simulink model "inv_rot_pen_RL_swingup_2_train"  (R2025b)
settings: Solver=FixedStepAuto  StartTime=0.0  StopTime=1  FixedStep=Ts  RelTol=1e-3
StopFcn:
  | myStopFcnAppendInitTime
values from neighbouring files (symbols this model uses):
  cfg = loaded.cfg    [continueFurutaMatlabSwingupTraining.m]    (also in evaluateFurutaController.m = makeFurutaConfig(); evaluateFurutaMatlabSwingupAgent.m = makeFurutaMatlabSwingupTD3Config(); finalizeFurutaDirectTD3Run.m = normalizeRunConfig(cfg, runDir); initFurutaSldrtHardwareWorkspace.m = makeFurutaMathWorksStyleWideTD3Config())
  i_max = 4    [initFurutaModelWorkspace.m]
  K = K_oben    [initFurutaModelWorkspace.m]
  Kp_i = db2mag(options.CurrentControllerKpDb)    [initFurutaModelWorkspace.m]    (also in initFurutaSldrtHardwareWorkspace.m = 2.5)
  omega0 = options.InitialOmega    [initFurutaModelWorkspace.m]
  param = get_parameter()    [initFurutaModelWorkspace.m]
  s = zpk("s")    [initFurutaModelWorkspace.m]    (also in initFurutaSldrtHardwareWorkspace.m)
  theta0 = options.InitialTheta    [initFurutaModelWorkspace.m]
  Tn_i = param.L / param.R    [initFurutaModelWorkspace.m]    (also in initFurutaSldrtHardwareWorkspace.m = 0.000286849073257)
undefined symbols (not defined in the file or in its folder): doneParams, rewardParams, safetyParams, X, Y, Z
libraries: sm_lib x19, nesl_utility x6, rllib x2, simulink x1
settings Model: SimulationMode=accelerator  Creator=abuj  LastModifiedBy=abuj
settings DataIOCC: SaveOutput=off  DSMLogging=off  SaveTime=off  ReturnWorkspaceOutputs=off
settings ExplorerConfigSet: SimMechanicsOpenEditorOnUpdate=off

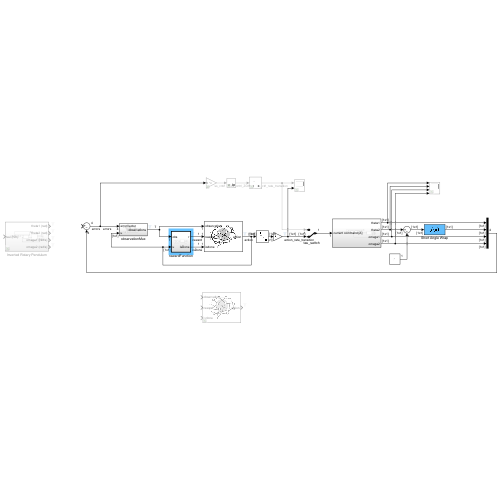
[thumbnail: Simulink's stored preview of the top-level diagram]
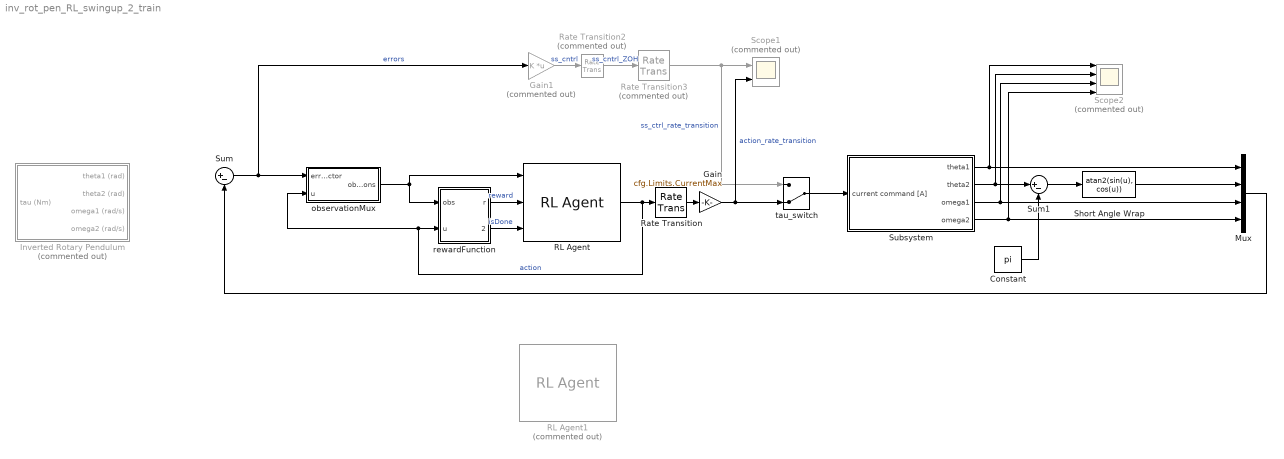
== system inv_rot_pen_RL_swingup_2_train ==
  Constant : Constant  Value=pi
  Gain : Gain  Gain=cfg.Limits.CurrentMax
  Gain1 : Gain  Commented=on  Gain=K  Multiplication=Matrix(K*u)
  Inverted Rotary Pendulum : Subsystem  Commented=on
  Mux : Mux
  RL Agent : rllib/RL Agent  Agent=agent  ExternalActionAsInput=off  ProvideLastAction=off  ProvideCumRwd=off  TreatAsDirectFeedthrough=on  UseStrictObservationDataTypes=off
  RL Agent1 : rllib/RL Agent  Commented=on  Agent=agent  ExternalActionAsInput=off  ProvideLastAction=off  ProvideCumRwd=off  TreatAsDirectFeedthrough=on  UseStrictObservationDataTypes=off
  Rate Transition : RateTransition  OutPortSampleTime=Ts
  Rate Transition2 : RateTransition  Commented=on  OutPortSampleTime=cfg.Agent.SampleTime
  Rate Transition3 : RateTransition  Commented=on  OutPortSampleTime=Ts
  Scope1 : Scope  Commented=on  NumInputPorts=2
      settings: ActiveDisplayYMinimum=-4.2971254580337988  ActiveDisplayYMaximum=0.512065850784593  DataLoggingVariableName=ScopeData4
  Scope2 : Scope  Commented=on  NumInputPorts=4
      settings: ActiveDisplayYMinimum=-1.667283029169482  ActiveDisplayYMaximum=0.18527228980949279
  Short Angle Wrap : Fcn  Expr=atan2(sin(u), cos(u))
  Subsystem : Subsystem
  Sum : Sum  Inputs=|+-
  Sum1 : Sum  Inputs=|+-
  observationMux : Subsystem
  rewardFunction : Subsystem  TreatAsAtomicUnit=on  SystemSampleTime=cfg.Agent.SampleTime
  tau_switch : ManualSwitch  CurrentSetting=0
  wires:
  Sum1/1 -> Short Angle Wrap/1
  Constant/1 -> Sum1/2
  Mux/1 -> Sum/2
  Rate Transition/1 -> Gain/1
  Subsystem/4(omega2) -> Scope2/4, Mux/4
  Subsystem/1(theta1) -> Scope2/1, Mux/1
  Subsystem/2(theta2) -> Scope2/2, Sum1/1
  Subsystem/3(omega1) -> Scope2/3, Mux/3
  Short Angle Wrap/1 -> Mux/2
  Gain1/1 -> Rate Transition2/1  "ss_cntrl"
  Rate Transition2/1 -> Rate Transition3/1  "ss_cntrl_ZOH"
  Rate Transition3/1 -> Scope1/1, tau_switch/1  "ss_ctrl_rate_transition"
  tau_switch/1 -> Subsystem/1(current command [A])
  Gain/1 -> Scope1/2, tau_switch/2  "action_rate_transition"
  rewardFunction/1(r) -> RL Agent/2  "reward"
  Sum/1 -> observationMux/1(errorVector), Gain1/1  "errors"
  rewardFunction/2(isDone) -> RL Agent/3  "isDone"
  RL Agent/1 -> rewardFunction/2(u), observationMux/2(u), Rate Transition/1  "action"
  observationMux/1(observations) -> rewardFunction/1(obs), RL Agent/1

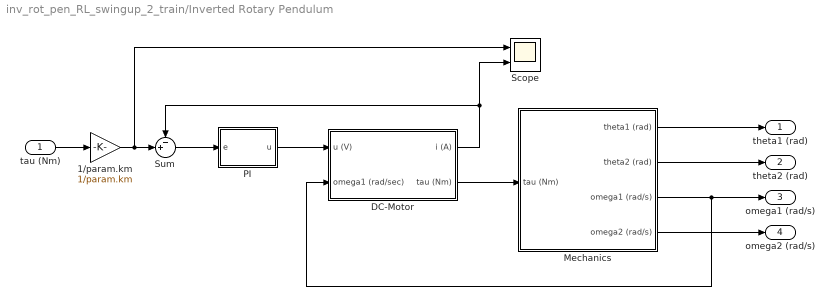
== system inv_rot_pen_RL_swingup_2_train/Inverted Rotary Pendulum ==
  tau (Nm) : Inport
  1/param.km : Gain  Gain=1/param.km
  DC-Motor : Subsystem
  Mechanics : Subsystem
  PI : Subsystem
  Scope : Scope  NumInputPorts=2
      settings: ActiveDisplayYMinimum=-0.091534229828850844  ActiveDisplayYMaximum=0.52735330073349629  DataLoggingVariableName=ScopeData2
  Sum : Sum  Inputs=-+|
  theta1 (rad) : Outport
  theta2 (rad) : Outport  Port=2
  omega1 (rad/s) : Outport  Port=3
  omega2 (rad/s) : Outport  Port=4
  wires:
  Mechanics/1(theta1 (rad)) -> theta1 (rad)/1
  Mechanics/2(theta2 (rad)) -> theta2 (rad)/1
  Mechanics/3(omega1 (rad/s)) -> DC-Motor/2(omega1 (rad/sec)), omega1 (rad/s)/1
  Mechanics/4(omega2 (rad/s)) -> omega2 (rad/s)/1
  DC-Motor/2(tau (Nm)) -> Mechanics/1(tau (Nm))
  Sum/1 -> PI/1(e)
  PI/1(u) -> DC-Motor/1(u (V))
  DC-Motor/1(i (A)) -> Scope/2, Sum/1
  tau (Nm)/1 -> 1/param.km/1
  1/param.km/1 -> Scope/1, Sum/2

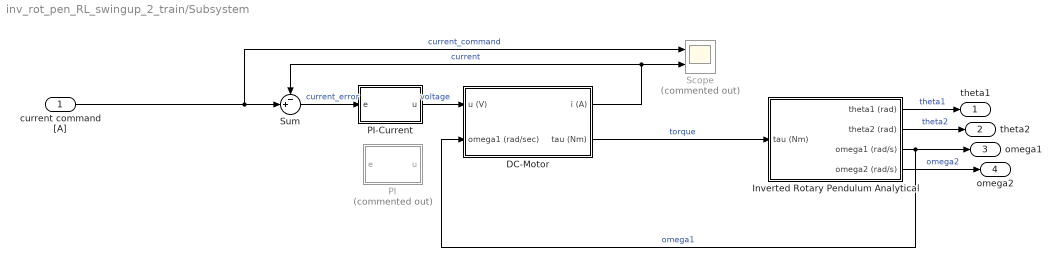
== system inv_rot_pen_RL_swingup_2_train/Subsystem ==
  current command [A] : Inport
  DC-Motor : Subsystem
  Inverted Rotary Pendulum Analytical : Subsystem
  PI : Subsystem  Commented=on
  PI-Current : Subsystem
  Scope : Scope  Commented=on  NumInputPorts=2
      settings: ActiveDisplayYMinimum=-4.5  ActiveDisplayYMaximum=0.49999999999999989
  Sum : Sum  Inputs=-+|
  theta1 : Outport
  theta2 : Outport  Port=2
  omega1 : Outport  Port=3
  omega2 : Outport  Port=4
  wires:
  Inverted Rotary Pendulum Analytical/3(omega1 (rad/s)) -> omega1/1, DC-Motor/2(omega1 (rad/sec))  "omega1"
  Inverted Rotary Pendulum Analytical/1(theta1 (rad)) -> theta1/1  "theta1"
  Inverted Rotary Pendulum Analytical/4(omega2 (rad/s)) -> omega2/1  "omega2"
  Inverted Rotary Pendulum Analytical/2(theta2 (rad)) -> theta2/1  "theta2"
  PI-Current/1(u) -> DC-Motor/1(u (V))  "voltage"
  DC-Motor/2(tau (Nm)) -> Inverted Rotary Pendulum Analytical/1(tau (Nm))  "torque"
  current command [A]/1 -> Scope/1, Sum/2  "current_command"
  DC-Motor/1(i (A)) -> Sum/1, Scope/2  "current"
  Sum/1 -> PI-Current/1(e)  "current_error"

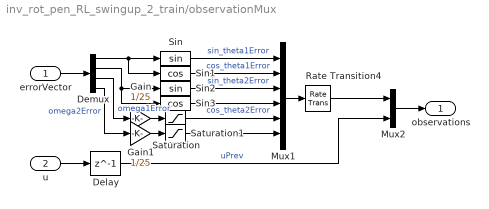
== system inv_rot_pen_RL_swingup_2_train/observationMux ==
  errorVector : Inport
  u : Inport  Port=2
  Delay : Delay  DelayLength=1
  Demux : Demux
  Gain : Gain  Gain=1/25
  Gain1 : Gain  Gain=1/25
  Mux1 : Mux  Inputs=6
  Mux2 : Mux  Inputs=2
  Rate Transition4 : RateTransition  OutPortSampleTime=cfg.Agent.SampleTime
  Saturation : Saturate  UpperLimit=25  LowerLimit=-25
  Saturation1 : Saturate  UpperLimit=25  LowerLimit=-25
  Sin : Trigonometry
  Sin1 : Trigonometry  Operator=cos
  Sin2 : Trigonometry
  Sin3 : Trigonometry  Operator=cos
  observations : Outport
  wires:
  Demux/2 -> Sin3/1, Sin2/1
  Sin1/1 -> Mux1/2  "cos_theta1Error"
  Demux/1 -> Sin1/1, Sin/1
  Rate Transition4/1 -> Mux2/1
  Mux1/1 -> Rate Transition4/1
  Sin/1 -> Mux1/1  "sin_theta1Error"
  Sin3/1 -> Mux1/4  "cos_theta2Error"
  errorVector/1 -> Demux/1
  Demux/4 -> Gain1/1  "omega2Error"
  Demux/3 -> Gain/1  "omega1Error"
  Sin2/1 -> Mux1/3  "sin_theta2Error"
  Mux2/1 -> observations/1
  u/1 -> Delay/1
  Delay/1 -> Mux2/2  "uPrev"
  Gain/1 -> Saturation/1
  Saturation/1 -> Mux1/5
  Gain1/1 -> Saturation1/1
  Saturation1/1 -> Mux1/6

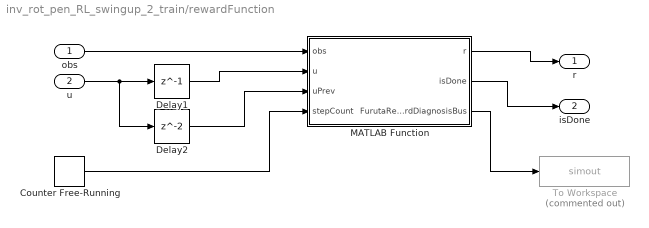
== system inv_rot_pen_RL_swingup_2_train/rewardFunction ==
  obs : Inport
  u : Inport  Port=2
  Counter Free-Running : simulink/Sources/Counter Free-Running  NumBits=16  tsamp=-1
  Delay1 : Delay  DelayLength=1  SampleTime=cfg.Agent.SampleTime
  Delay2 : Delay  SampleTime=cfg.Agent.SampleTime
  MATLAB Function : MATLAB Function  TreatAsAtomicUnit=on
  To Workspace : ToWorkspace  Commented=on  VariableName=simout  SaveFormat=Timeseries  SampleTime=-1
  r : Outport
  isDone : Outport  Port=2
  wires:
  MATLAB Function/2(isDone) -> isDone/1
  obs/1 -> MATLAB Function/1(obs)
  MATLAB Function/1(r) -> r/1
  u/1 -> Delay2/1, Delay1/1
  Delay2/1 -> MATLAB Function/3(uPrev)
  Delay1/1 -> MATLAB Function/2(u)
  MATLAB Function/3(FurutaRewardDiagnosisBus) -> To Workspace/1
  Counter Free-Running/1 -> MATLAB Function/4(stepCount)

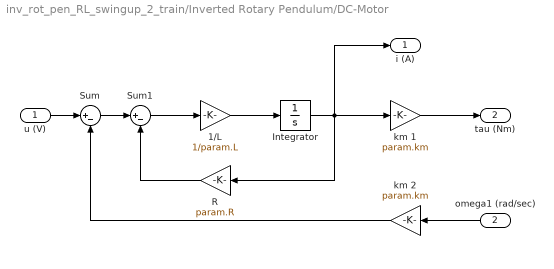
== system inv_rot_pen_RL_swingup_2_train/Inverted Rotary Pendulum/DC-Motor ==
  u (V) : Inport
  omega1 (rad/sec) : Inport  Port=2
  1/L : Gain  Gain=1/param.L
  Integrator : Integrator
  R : Gain  Gain=param.R
  Sum : Sum  Inputs=|+-
  Sum1 : Sum  Inputs=|+-
  km 1 : Gain  Gain=param.km
  km 2 : Gain  Gain=param.km
  i (A) : Outport
  tau (Nm) : Outport  Port=2
  wires:
  R/1 -> Sum1/2
  Integrator/1 -> i (A)/1, km 1/1, R/1
  u (V)/1 -> Sum/1
  Sum1/1 -> 1/L/1
  Sum/1 -> Sum1/1
  1/L/1 -> Integrator/1
  omega1 (rad/sec)/1 -> km 2/1
  km 2/1 -> Sum/2
  km 1/1 -> tau (Nm)/1

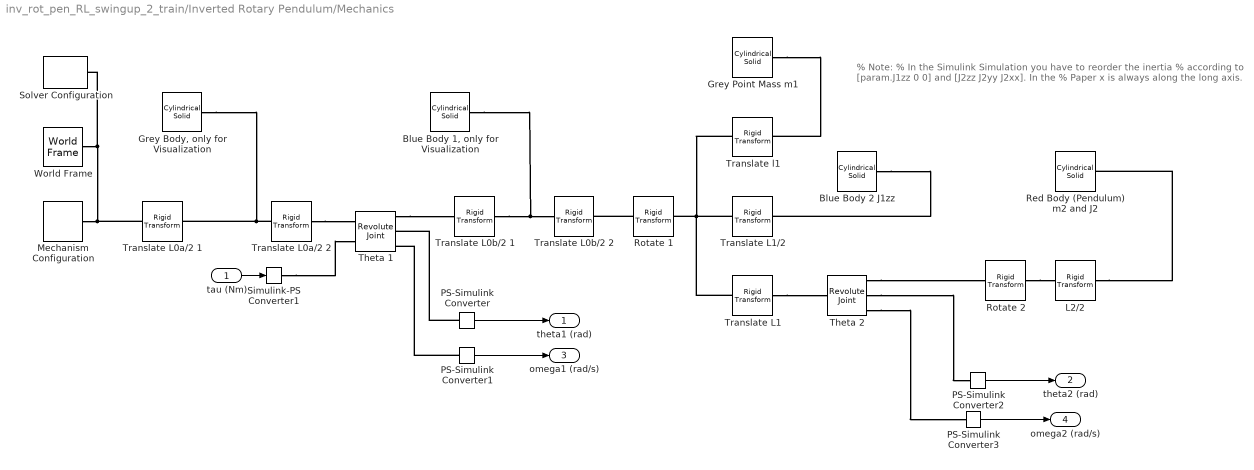
== system inv_rot_pen_RL_swingup_2_train/Inverted Rotary Pendulum/Mechanics ==
  note: % Note:
      | % In the Simulink Simulation you have to reorder the inertia
      | % according to [param.J1zz 0 0] and [J2zz J2yy J2xx]. In the
      | % Paper x is always along the long axis.
  tau (Nm) : Inport
  "Blue Body 1, only for Visualization" : sm_lib/Body Elements/Cylindrical Solid  CylinderRadius=param.r0b  CylinderRadiusUnits=m  CylinderLength=param.L0b  CylinderLengthUnits=m  ExportEntireGeometry=off  InertiaType=PointMass  BasedOnType=Density  Density=1000  DensityUnits=kg/m^3  Mass=0  MassUnits=kg  CenterOfMass=[0 0 0]  CenterOfMassUnits=m  MomentsOfInertia=[0 0 0]  MomentsOfInertiaUnits=kg*m^2  ProductsOfInertia=[0 0 0]  ProductsOfInertiaUnits=kg*m^2  GraphicType=FromGeometry  MarkerShape=Sphere  MarkerSize=10  GraphicVisPropType=SimpleVisualProperties  GraphicDiffuseColor=[0.0 0.6 1.0]  GraphicOpacity=1  GraphicSpecularColor=[0.5 0.5 0.5 1.0]  GraphicAmbientColor=[0.15 0.15 0.15 1.0]  GraphicEmissiveColor=[0.0 0.0 0.0 1.0]  GraphicShininess=75  DoExposeReferenceFrame=on  SerializedFrames=<Frames/>
  Blue Body 2 J1zz : sm_lib/Body Elements/Cylindrical Solid  CylinderRadius=param.r1  CylinderRadiusUnits=m  CylinderLength=param.L1  CylinderLengthUnits=m  ExportEntireGeometry=off  InertiaType=Custom  BasedOnType=Density  Density=1000  DensityUnits=kg/m^3  Mass=0  MassUnits=kg  CenterOfMass=[0 0 0]  CenterOfMassUnits=m  MomentsOfInertia=[param.J1zz 0 0]  MomentsOfInertiaUnits=kg*m^2  ProductsOfInertia=[0 0 0]  ProductsOfInertiaUnits=kg*m^2  GraphicType=FromGeometry  MarkerShape=Sphere  MarkerSize=10  GraphicVisPropType=SimpleVisualProperties  GraphicDiffuseColor=[0.0 0.6 1.0]  GraphicOpacity=1  GraphicSpecularColor=[0.5 0.5 0.5 1.0]  GraphicAmbientColor=[0.15 0.15 0.15 1.0]  GraphicEmissiveColor=[0.0 0.0 0.0 1.0]  GraphicShininess=75  DoExposeReferenceFrame=on  SerializedFrames=<Frames/>
  "Grey Body, only for Visualization" : sm_lib/Body Elements/Cylindrical Solid  CylinderRadius=param.r0a  CylinderRadiusUnits=m  CylinderLength=param.L0a  CylinderLengthUnits=m  ExportEntireGeometry=off  InertiaType=PointMass  BasedOnType=Density  Density=1000  DensityUnits=kg/m^3  Mass=0  MassUnits=kg  CenterOfMass=[0 0 0]  CenterOfMassUnits=m  MomentsOfInertia=[0 0 0]  MomentsOfInertiaUnits=kg*m^2  ProductsOfInertia=[0 0 0]  ProductsOfInertiaUnits=kg*m^2  GraphicType=FromGeometry  MarkerShape=Sphere  MarkerSize=10  GraphicVisPropType=SimpleVisualProperties  GraphicDiffuseColor=[0.5 0.5 0.5]  GraphicOpacity=1  GraphicSpecularColor=[0.5 0.5 0.5 1.0]  GraphicAmbientColor=[0.15 0.15 0.15 1.0]  GraphicEmissiveColor=[0.0 0.0 0.0 1.0]  GraphicShininess=75  DoExposeReferenceFrame=on  SerializedFrames=<Frames/>
  Grey Point Mass m1 : sm_lib/Body Elements/Cylindrical Solid  CylinderRadius=1  CylinderRadiusUnits=m  CylinderLength=1  CylinderLengthUnits=m  ExportEntireGeometry=off  InertiaType=PointMass  BasedOnType=Density  Density=1000  DensityUnits=kg/m^3  Mass=param.m1  MassUnits=kg  CenterOfMass=[0 0 0]  CenterOfMassUnits=m  MomentsOfInertia=[1 1 1]  MomentsOfInertiaUnits=kg*m^2  ProductsOfInertia=[0 0 0]  ProductsOfInertiaUnits=kg*m^2  GraphicType=Marker  MarkerShape=Sphere  MarkerSize=10  GraphicVisPropType=SimpleVisualProperties  GraphicDiffuseColor=[0.5 0.5 0.5]  GraphicOpacity=1  GraphicSpecularColor=[0.5 0.5 0.5 1.0]  GraphicAmbientColor=[0.15 0.15 0.15 1.0]  GraphicEmissiveColor=[0.0 0.0 0.0 1.0]  GraphicShininess=75  DoExposeReferenceFrame=on  SerializedFrames=<Frames/>
  L2/2 : sm_lib/Frames and Transforms/Rigid Transform  RotationMethod=None  FollAlignAxisA=+X  BaseAlignAxisA=+Y  FollAlignAxisB=+Y  BaseAlignAxisB=+Z  RotationStandardAxis=+Z  RotationAngle=0  RotationAngleUnits=deg  RotationArbitraryAxis=[0 0 1]  RotationSequenceAxes=FollowerAxes  RotationSequence=ZYX  RotationSequenceAngles=[0 pi/2 0]  RotationSequenceAnglesUnits=rad  RotationMatrix=[1 0 0;0 1 0;0 0 1]  Quaternion=[1 0 0 0]  TranslationMethod=Cartesian  TranslationCartesianOffset=[0 0 param.L2/2]  TranslationCartesianOffsetUnits=m  TranslationStandardAxis=+Z  TranslationStandardOffset=0  TranslationStandardOffsetUnits=m  TranslationROffset=0  TranslationROffsetUnits=m  TranslationThetaOffset=0  TranslationThetaOffsetUnits=deg  TranslationZOffset=0  TranslationZOffsetUnits=m
  Mechanism Configuration : sm_lib/Utilities/Mechanism Configuration  UniformGravity=Constant  GravityVector=[0 0 -param.g]  GravityVectorUnits=m/s^2  LinearizationDelta=0.001  JointModeTransitionNonlinearIterations=2
  PS-Simulink Converter{,1..3} (4 alike) : nesl_utility/PS-Simulink Converter  PhysicalDomain=network_engine_domain  SubClassName=ps_output  LeftPortType=input  RightPortType=output  PseudoPeriodic=off  Frequencies=[]  VectorFormat=inherit  Unit=inherit  AffineConversion=off
  Red Body (Pendulum) m2 and J2 : sm_lib/Body Elements/Cylindrical Solid  CylinderRadius=param.r2  CylinderRadiusUnits=m  CylinderLength=param.L2  CylinderLengthUnits=m  ExportEntireGeometry=off  InertiaType=Custom  BasedOnType=Density  Density=1000  DensityUnits=kg/m^3  Mass=param.m2  MassUnits=kg  CenterOfMass=[0 0 0]  CenterOfMassUnits=m  MomentsOfInertia=[param.J2zz param.J2yy param.J2xx]  MomentsOfInertiaUnits=kg*m^2  ProductsOfInertia=[0 0 0]  ProductsOfInertiaUnits=kg*m^2  GraphicType=FromGeometry  MarkerShape=Sphere  MarkerSize=10  GraphicVisPropType=SimpleVisualProperties  GraphicDiffuseColor=[1.0 0.2 0.2]  GraphicOpacity=1  GraphicSpecularColor=[0.5 0.5 0.5 1.0]  GraphicAmbientColor=[0.15 0.15 0.15 1.0]  GraphicEmissiveColor=[0.0 0.0 0.0 1.0]  GraphicShininess=75  DoExposeReferenceFrame=on  SerializedFrames=<Frames/>
  Rotate 1 : sm_lib/Frames and Transforms/Rigid Transform  RotationMethod=RotationSequence  FollAlignAxisA=+X  BaseAlignAxisA=+Y  FollAlignAxisB=+Y  BaseAlignAxisB=+Z  RotationStandardAxis=+Z  RotationAngle=0  RotationAngleUnits=deg  RotationArbitraryAxis=[0 0 1]  RotationSequenceAxes=FollowerAxes  RotationSequence=ZYX  RotationSequenceAngles=[0 pi/2 0]  RotationSequenceAnglesUnits=rad  RotationMatrix=[1 0 0;0 1 0;0 0 1]  Quaternion=[1 0 0 0]  TranslationMethod=None  TranslationCartesianOffset=[0 0 0]  TranslationCartesianOffsetUnits=m  TranslationStandardAxis=+Z  TranslationStandardOffset=0  TranslationStandardOffsetUnits=m  TranslationROffset=0  TranslationROffsetUnits=m  TranslationThetaOffset=0  TranslationThetaOffsetUnits=deg  TranslationZOffset=0  TranslationZOffsetUnits=m
  Rotate 2 : sm_lib/Frames and Transforms/Rigid Transform  RotationMethod=RotationSequence  FollAlignAxisA=+X  BaseAlignAxisA=+Y  FollAlignAxisB=+Y  BaseAlignAxisB=+Z  RotationStandardAxis=+Z  RotationAngle=0  RotationAngleUnits=deg  RotationArbitraryAxis=[0 0 1]  RotationSequenceAxes=FollowerAxes  RotationSequence=ZYX  RotationSequenceAngles=[0 pi/2 0]  RotationSequenceAnglesUnits=rad  RotationMatrix=[1 0 0;0 1 0;0 0 1]  Quaternion=[1 0 0 0]  TranslationMethod=None  TranslationCartesianOffset=[0 0 0]  TranslationCartesianOffsetUnits=m  TranslationStandardAxis=+Z  TranslationStandardOffset=0  TranslationStandardOffsetUnits=m  TranslationROffset=0  TranslationROffsetUnits=m  TranslationThetaOffset=0  TranslationThetaOffsetUnits=deg  TranslationZOffset=0  TranslationZOffsetUnits=m
  Simulink-PS Converter1 : nesl_utility/Simulink-PS Converter  PhysicalDomain=network_engine_domain  SubClassName=ps_input  LeftPortType=input  RightPortType=output  PseudoPeriodic=off  Frequencies=[]  NoiseDistribution=none  NoiseParameters=[]  Unit=1  AffineConversion=off  FilteringAndDerivatives=provide  SimscapeFilterOrder=1  InputFilterTimeConstant=0.001  UdotUserProvided=0
  Solver Configuration : nesl_utility/Solver Configuration  PhysicalDomain=network_engine_domain  SubClassName=solver  LeftPortType=input  RightPortType=generic  Tones=[]  Harmonics=[]  SimulateNoise=off  Profile=off  UseLocalSampling=off  EnableSwitchedLinearOptims=on  FrequencyDomain=off  UseCCode=off  RelTol=0.001  AbsTol=0.001  MinStep=1e-09  ToWorkspace=off  RevertToSquareIcSolve=off  NumHomotopyIterations=100  PhasorMode=off  PhasorModeNumHarmonics=1  ConsistencySolver=NEWTON_XTOL_AFTER_FTOL  IndexReductionMethod=DerivativeReplacement  DoDC=off  ResidualTolerance=1e-09  ConsistencyTolSource=GLOBAL  ConsistencyAbsTol=0.001  ConsistencyRelTol=0.001  ConsistencyTolFactor=0.001  UseLocalSolver=off  LocalSolverChoice=NE_BACKWARD_EULER_ADVANCER  ResolveIndetEquations=on  FunctionEvalNumThread=1  LocalSolverSampleTime=0.001  DoFixedCost=off  MaxNonlinIter=3  MaxModeIter=2  ComputeImpulses=off  ImpulseIterations=2  LinearAlgebra=auto  LinearAlgebraNumThread=0  EquationFormulation=NE_TIME_EF  DelaysMemoryBudget=1024  AutomaticFiltering=on  FilteringTimeConstant=0.001  PartitionStorageMethod=AS_NEEDED  PartitionMemoryBudget=1024  PartitionMethod=ROBUST  MultibodyUseLocalSolver=off  MultibodyLocalSolverChoice=ODE1  MultibodyLocalSolverSampleTime=0.001
  Theta 1 : sm_lib/Joints/Revolute Joint  JointMode=Normal  CompositeWrenchDir=FollowerOnBase  CompositeWrenchFrame=BaseFrame  SenseConstraintForce=off  SenseConstraintTorque=off  SenseTotalForce=off  SenseTotalTorque=off  PositionTargetSpecify=on  PositionTargetPriority=High  PositionTargetValue=theta0(1)  PositionTargetValueUnits=rad  VelocityTargetSpecify=off  VelocityTargetPriority=High  VelocityTargetValue=0  VelocityTargetValueUnits=deg/s  EquilibriumPosition=0  EquilibriumPositionUnits=rad  SpringStiffness=0  SpringStiffnessUnits=N*m/rad  DampingCoefficient=param.b1  DampingCoefficientUnits=N*m*s/rad  LowerLimitSpecify=off  LowerLimitBound=-90  LowerLimitBoundUnits=deg  LowerLimitStiffness=1e4  LowerLimitStiffnessUnits=N*m/deg  LowerLimitDamping=10  LowerLimitDampingUnits=N*m/(deg/s)  LowerLimitTransitionRegionWidth=0.1  LowerLimitTransitionRegionWidthUnits=deg  UpperLimitSpecify=off  UpperLimitBound=90  UpperLimitBoundUnits=deg  UpperLimitStiffness=1e4  UpperLimitStiffnessUnits=N*m/deg  UpperLimitDamping=10  UpperLimitDampingUnits=N*m/(deg/s)  UpperLimitTransitionRegionWidth=0.1  UpperLimitTransitionRegionWidthUnits=deg  TorqueActuationMode=InputTorque  MotionActuationMode=ComputedMotion  SensePosition=on  SenseVelocity=on  SenseAcceleration=off  SenseTorqueForce=off  SenseLowerLimitTorqueForce=off  SenseUpperLimitTorqueForce=off
  Theta 2 : sm_lib/Joints/Revolute Joint  JointMode=Normal  CompositeWrenchDir=FollowerOnBase  CompositeWrenchFrame=BaseFrame  SenseConstraintForce=off  SenseConstraintTorque=off  SenseTotalForce=off  SenseTotalTorque=off  PositionTargetSpecify=on  PositionTargetPriority=High  PositionTargetValue=theta0(2)  PositionTargetValueUnits=rad  VelocityTargetSpecify=off  VelocityTargetPriority=High  VelocityTargetValue=0  VelocityTargetValueUnits=deg/s  EquilibriumPosition=0  EquilibriumPositionUnits=rad  SpringStiffness=0  SpringStiffnessUnits=N*m/rad  DampingCoefficient=param.b2  DampingCoefficientUnits=N*m*s/rad  LowerLimitSpecify=off  LowerLimitBound=-90  LowerLimitBoundUnits=deg  LowerLimitStiffness=1e4  LowerLimitStiffnessUnits=N*m/deg  LowerLimitDamping=10  LowerLimitDampingUnits=N*m/(deg/s)  LowerLimitTransitionRegionWidth=0.1  LowerLimitTransitionRegionWidthUnits=deg  UpperLimitSpecify=off  UpperLimitBound=90  UpperLimitBoundUnits=deg  UpperLimitStiffness=1e4  UpperLimitStiffnessUnits=N*m/deg  UpperLimitDamping=10  UpperLimitDampingUnits=N*m/(deg/s)  UpperLimitTransitionRegionWidth=0.1  UpperLimitTransitionRegionWidthUnits=deg  TorqueActuationMode=NoTorque  MotionActuationMode=ComputedMotion  SensePosition=on  SenseVelocity=on  SenseAcceleration=off  SenseTorqueForce=off  SenseLowerLimitTorqueForce=off  SenseUpperLimitTorqueForce=off
  Translate L0a/2 1 : sm_lib/Frames and Transforms/Rigid Transform  RotationMethod=None  FollAlignAxisA=+X  BaseAlignAxisA=+Y  FollAlignAxisB=+Y  BaseAlignAxisB=+Z  RotationStandardAxis=+Z  RotationAngle=0  RotationAngleUnits=deg  RotationArbitraryAxis=[0 0 1]  RotationSequenceAxes=FollowerAxes  RotationSequence=ZYX  RotationSequenceAngles=[0 0 0]  RotationSequenceAnglesUnits=rad  RotationMatrix=[1 0 0;0 1 0;0 0 1]  Quaternion=[1 0 0 0]  TranslationMethod=Cartesian  TranslationCartesianOffset=[0 0 param.L0a/2]  TranslationCartesianOffsetUnits=m  TranslationStandardAxis=+Z  TranslationStandardOffset=0  TranslationStandardOffsetUnits=m  TranslationROffset=0  TranslationROffsetUnits=m  TranslationThetaOffset=0  TranslationThetaOffsetUnits=deg  TranslationZOffset=0  TranslationZOffsetUnits=m
  Translate L0a/2 2 : sm_lib/Frames and Transforms/Rigid Transform  RotationMethod=None  FollAlignAxisA=+X  BaseAlignAxisA=+Y  FollAlignAxisB=+Y  BaseAlignAxisB=+Z  RotationStandardAxis=+Z  RotationAngle=0  RotationAngleUnits=deg  RotationArbitraryAxis=[0 0 1]  RotationSequenceAxes=FollowerAxes  RotationSequence=ZYX  RotationSequenceAngles=[0 0 0]  RotationSequenceAnglesUnits=rad  RotationMatrix=[1 0 0;0 1 0;0 0 1]  Quaternion=[1 0 0 0]  TranslationMethod=Cartesian  TranslationCartesianOffset=[0 0 param.L0a/2]  TranslationCartesianOffsetUnits=m  TranslationStandardAxis=+Z  TranslationStandardOffset=0  TranslationStandardOffsetUnits=m  TranslationROffset=0  TranslationROffsetUnits=m  TranslationThetaOffset=0  TranslationThetaOffsetUnits=deg  TranslationZOffset=0  TranslationZOffsetUnits=m
  Translate L0b/2 1 : sm_lib/Frames and Transforms/Rigid Transform  RotationMethod=None  FollAlignAxisA=+X  BaseAlignAxisA=+Y  FollAlignAxisB=+Y  BaseAlignAxisB=+Z  RotationStandardAxis=+Z  RotationAngle=0  RotationAngleUnits=deg  RotationArbitraryAxis=[0 0 1]  RotationSequenceAxes=FollowerAxes  RotationSequence=ZYX  RotationSequenceAngles=[0 0 0]  RotationSequenceAnglesUnits=rad  RotationMatrix=[1 0 0;0 1 0;0 0 1]  Quaternion=[1 0 0 0]  TranslationMethod=Cartesian  TranslationCartesianOffset=[0 0 param.L0b/2]  TranslationCartesianOffsetUnits=m  TranslationStandardAxis=+Z  TranslationStandardOffset=0  TranslationStandardOffsetUnits=m  TranslationROffset=0  TranslationROffsetUnits=m  TranslationThetaOffset=0  TranslationThetaOffsetUnits=deg  TranslationZOffset=0  TranslationZOffsetUnits=m
  Translate L0b/2 2 : sm_lib/Frames and Transforms/Rigid Transform  RotationMethod=None  FollAlignAxisA=+X  BaseAlignAxisA=+Y  FollAlignAxisB=+Y  BaseAlignAxisB=+Z  RotationStandardAxis=+Z  RotationAngle=0  RotationAngleUnits=deg  RotationArbitraryAxis=[0 0 1]  RotationSequenceAxes=FollowerAxes  RotationSequence=ZYX  RotationSequenceAngles=[0 0 0]  RotationSequenceAnglesUnits=rad  RotationMatrix=[1 0 0;0 1 0;0 0 1]  Quaternion=[1 0 0 0]  TranslationMethod=Cartesian  TranslationCartesianOffset=[0 0 param.L0b/2]  TranslationCartesianOffsetUnits=m  TranslationStandardAxis=+Z  TranslationStandardOffset=0  TranslationStandardOffsetUnits=m  TranslationROffset=0  TranslationROffsetUnits=m  TranslationThetaOffset=0  TranslationThetaOffsetUnits=deg  TranslationZOffset=0  TranslationZOffsetUnits=m
  Translate L1 : sm_lib/Frames and Transforms/Rigid Transform  RotationMethod=None  FollAlignAxisA=+X  BaseAlignAxisA=+Y  FollAlignAxisB=+Y  BaseAlignAxisB=+Z  RotationStandardAxis=+Z  RotationAngle=0  RotationAngleUnits=deg  RotationArbitraryAxis=[0 0 1]  RotationSequenceAxes=FollowerAxes  RotationSequence=ZYX  RotationSequenceAngles=[0 0 0]  RotationSequenceAnglesUnits=rad  RotationMatrix=[1 0 0;0 1 0;0 0 1]  Quaternion=[1 0 0 0]  TranslationMethod=Cartesian  TranslationCartesianOffset=[0 0 param.L1]  TranslationCartesianOffsetUnits=m  TranslationStandardAxis=+Z  TranslationStandardOffset=0  TranslationStandardOffsetUnits=m  TranslationROffset=0  TranslationROffsetUnits=m  TranslationThetaOffset=0  TranslationThetaOffsetUnits=deg  TranslationZOffset=0  TranslationZOffsetUnits=m
  Translate L1/2 : sm_lib/Frames and Transforms/Rigid Transform  RotationMethod=None  FollAlignAxisA=+X  BaseAlignAxisA=+Y  FollAlignAxisB=+Y  BaseAlignAxisB=+Z  RotationStandardAxis=+Z  RotationAngle=0  RotationAngleUnits=deg  RotationArbitraryAxis=[0 0 1]  RotationSequenceAxes=FollowerAxes  RotationSequence=ZYX  RotationSequenceAngles=[0 0 0]  RotationSequenceAnglesUnits=rad  RotationMatrix=[1 0 0;0 1 0;0 0 1]  Quaternion=[1 0 0 0]  TranslationMethod=Cartesian  TranslationCartesianOffset=[0 0 param.L1/2]  TranslationCartesianOffsetUnits=m  TranslationStandardAxis=+Z  TranslationStandardOffset=0  TranslationStandardOffsetUnits=m  TranslationROffset=0  TranslationROffsetUnits=m  TranslationThetaOffset=0  TranslationThetaOffsetUnits=deg  TranslationZOffset=0  TranslationZOffsetUnits=m
  Translate l1 : sm_lib/Frames and Transforms/Rigid Transform  RotationMethod=None  FollAlignAxisA=+X  BaseAlignAxisA=+Y  FollAlignAxisB=+Y  BaseAlignAxisB=+Z  RotationStandardAxis=+Z  RotationAngle=0  RotationAngleUnits=deg  RotationArbitraryAxis=[0 0 1]  RotationSequenceAxes=FollowerAxes  RotationSequence=ZYX  RotationSequenceAngles=[0 0 0]  RotationSequenceAnglesUnits=rad  RotationMatrix=[1 0 0;0 1 0;0 0 1]  Quaternion=[1 0 0 0]  TranslationMethod=Cartesian  TranslationCartesianOffset=[0 0 param.l1]  TranslationCartesianOffsetUnits=m  TranslationStandardAxis=+Z  TranslationStandardOffset=0  TranslationStandardOffsetUnits=m  TranslationROffset=0  TranslationROffsetUnits=m  TranslationThetaOffset=0  TranslationThetaOffsetUnits=deg  TranslationZOffset=0  TranslationZOffsetUnits=m
  World Frame : sm_lib/Frames and Transforms/World Frame
  theta1 (rad) : Outport
  theta2 (rad) : Outport  Port=2
  omega1 (rad/s) : Outport  Port=3
  omega2 (rad/s) : Outport  Port=4
  wires:
  PS-Simulink Converter2/1 -> theta2 (rad)/1
  PS-Simulink Converter1/1 -> omega1 (rad/s)/1
  PS-Simulink Converter3/1 -> omega2 (rad/s)/1
  tau (Nm)/1 -> Simulink-PS Converter1/1
  PS-Simulink Converter/1 -> theta1 (rad)/1
  connections:
  PS-Simulink Converter1/LConn1 -- Theta 1/RConn3
  Rotate 1/LConn1 -- Translate L0b/2 2/RConn1
  Translate L1/RConn1 -- Theta 2/LConn1
  World Frame/RConn1 -- Translate L0a/2 1/LConn1 -- Mechanism Configuration/RConn1 -- Solver Configuration/RConn1
  Rotate 2/RConn1 -- L2/2/LConn1
  Translate L0a/2 2/LConn1 -- "Grey Body, only for Visualization"/RConn1 -- Translate L0a/2 1/RConn1
  Theta 2/RConn3 -- PS-Simulink Converter3/LConn1
  Theta 2/RConn2 -- PS-Simulink Converter2/LConn1
  Translate L0b/2 1/RConn1 -- "Blue Body 1, only for Visualization"/RConn1 -- Translate L0b/2 2/LConn1
  Theta 1/RConn1 -- Translate L0b/2 1/LConn1
  PS-Simulink Converter/LConn1 -- Theta 1/RConn2
  Translate l1/LConn1 -- Translate L1/2/LConn1 -- Translate L1/LConn1 -- Rotate 1/RConn1
  Blue Body 2 J1zz/RConn1 -- Translate L1/2/RConn1
  Simulink-PS Converter1/RConn1 -- Theta 1/LConn2
  Translate L0a/2 2/RConn1 -- Theta 1/LConn1
  Theta 2/RConn1 -- Rotate 2/LConn1
  Grey Point Mass m1/RConn1 -- Translate l1/RConn1
  L2/2/RConn1 -- Red Body (Pendulum) m2 and J2/RConn1

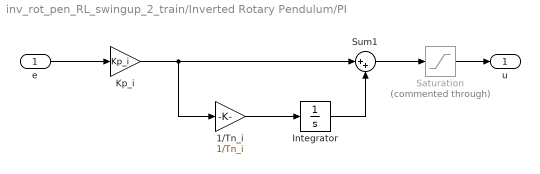
== system inv_rot_pen_RL_swingup_2_train/Inverted Rotary Pendulum/PI ==
  e : Inport
  1/Tn_i : Gain  Gain=1/Tn_i
  Integrator : Integrator  UpperSaturationLimit=i_max  LowerSaturationLimit=-i_max
  Kp_i : Gain  Gain=Kp_i
  Saturation : Saturate  Commented=through  UpperLimit=i_max  LowerLimit=-i_max
  Sum1 : Sum  Inputs=|++
  u : Outport
  wires:
  Integrator/1 -> Sum1/2
  Sum1/1 -> Saturation/1
  Kp_i/1 -> Sum1/1, 1/Tn_i/1
  1/Tn_i/1 -> Integrator/1
  e/1 -> Kp_i/1
  Saturation/1 -> u/1

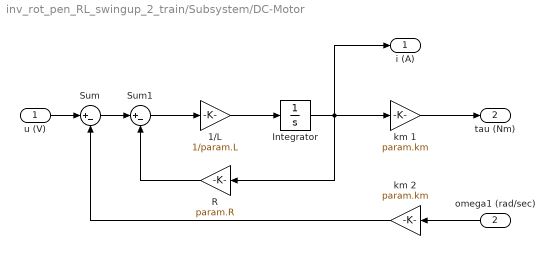
== system inv_rot_pen_RL_swingup_2_train/Subsystem/DC-Motor ==
  u (V) : Inport
  omega1 (rad/sec) : Inport  Port=2
  1/L : Gain  Gain=1/param.L
  Integrator : Integrator
  R : Gain  Gain=param.R
  Sum : Sum  Inputs=|+-
  Sum1 : Sum  Inputs=|+-
  km 1 : Gain  Gain=param.km
  km 2 : Gain  Gain=param.km
  i (A) : Outport
  tau (Nm) : Outport  Port=2
  wires:
  R/1 -> Sum1/2
  Integrator/1 -> i (A)/1, km 1/1, R/1
  u (V)/1 -> Sum/1
  Sum1/1 -> 1/L/1
  Sum/1 -> Sum1/1
  1/L/1 -> Integrator/1
  omega1 (rad/sec)/1 -> km 2/1
  km 2/1 -> Sum/2
  km 1/1 -> tau (Nm)/1

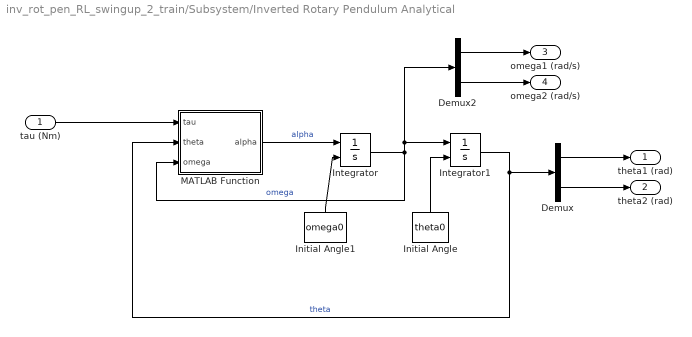
== system inv_rot_pen_RL_swingup_2_train/Subsystem/Inverted Rotary Pendulum Analytical ==
  tau (Nm) : Inport
  Demux : Demux  Outputs=2
  Demux2 : Demux  Outputs=2
  Initial Angle : Constant  Value=theta0
  Initial Angle1 : Constant  Value=omega0
  Integrator : Integrator  InitialConditionSource=external
  Integrator1 : Integrator  InitialConditionSource=external  InitialCondition=[0.1;0]
  MATLAB Function : MATLAB Function  TreatAsAtomicUnit=on
  theta1 (rad) : Outport
  theta2 (rad) : Outport  Port=2
  omega1 (rad/s) : Outport  Port=3
  omega2 (rad/s) : Outport  Port=4
  wires:
  Demux/2 -> theta2 (rad)/1
  MATLAB Function/1(alpha) -> Integrator/1  "alpha"
  tau (Nm)/1 -> MATLAB Function/1(tau)
  Integrator1/1 -> MATLAB Function/2(theta), Demux/1  "theta"
  Demux/1 -> theta1 (rad)/1
  Integrator/1 -> Demux2/1, Integrator1/1, MATLAB Function/3(omega)  "omega"
  Demux2/1 -> omega1 (rad/s)/1
  Initial Angle/1 -> Integrator1/2
  Demux2/2 -> omega2 (rad/s)/1
  Initial Angle1/1 -> Integrator/2

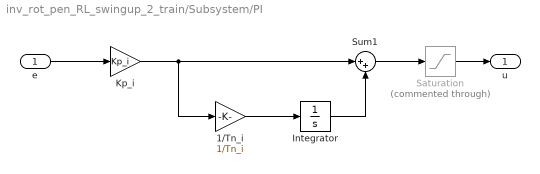
== system inv_rot_pen_RL_swingup_2_train/Subsystem/PI ==
  e : Inport
  1/Tn_i : Gain  Gain=1/Tn_i
  Integrator : Integrator  UpperSaturationLimit=i_max  LowerSaturationLimit=-i_max
  Kp_i : Gain  Gain=Kp_i
  Saturation : Saturate  Commented=through  UpperLimit=i_max  LowerLimit=-i_max
  Sum1 : Sum  Inputs=|++
  u : Outport
  wires:
  Integrator/1 -> Sum1/2
  Sum1/1 -> Saturation/1
  Kp_i/1 -> Sum1/1, 1/Tn_i/1
  1/Tn_i/1 -> Integrator/1
  e/1 -> Kp_i/1
  Saturation/1 -> u/1

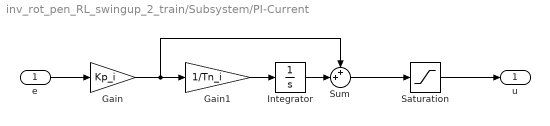
== system inv_rot_pen_RL_swingup_2_train/Subsystem/PI-Current ==
  e : Inport
  Gain : Gain  Gain=Kp_i
  Gain1 : Gain  Gain=1/Tn_i
  Integrator : Integrator  LimitOutput=on  UpperSaturationLimit=cfg.Limits.VoltageMax  LowerSaturationLimit=-cfg.Limits.VoltageMax
  Saturation : Saturate  UpperLimit=cfg.Limits.VoltageMax  LowerLimit=-cfg.Limits.VoltageMax
  Sum : Sum  Inputs=++|
  u : Outport
  wires:
  Gain1/1 -> Integrator/1
  e/1 -> Gain/1
  Integrator/1 -> Sum/2
  Gain/1 -> Gain1/1, Sum/1
  Sum/1 -> Saturation/1
  Saturation/1 -> u/1

== matlab function inv_rot_pen_RL_swingup_2_train/Subsystem/Inverted Rotary Pendulum Analytical/MATLAB Function ==
  data: tau input size=1; alpha output size=[2,1]; theta input size=[2,1]; omega input size=[2,1]; param parameter
function alpha = fcn(tau, theta, omega, param)

    % M(q) * qdd + C(q,qdot) * qdot + G(q) + D * qdot = tau
    [M, C, G, D] = calculate_dynamics_furuta(theta, omega, param);
    alpha = M \ ( [tau; 0] - (C + D) * omega - G );

end

== matlab function inv_rot_pen_RL_swingup_2_train/rewardFunction/MATLAB Function ==
  data: obs input; u input; uPrev input; stepCount input; rewardParams parameter; doneParams parameter; r output; isDone output; safetyParams parameter; FurutaRewardDiagnosisBus output Bus: FurutaRewardDiagnosisBus
function [r, isDone, FurutaRewardDiagnosisBus] = fcn(obs, u, uPrev, stepCount, rewardParams, doneParams, safetyParams)
% params declared as block Parameter via Ports & Data Manager

[r, FurutaRewardDiagnosisBus] = rewardFcnFurutaSwingupCapture( ...
    obs, u, uPrev, stepCount, rewardParams, safetyParams);

isDone = isDoneFcnFurutaSwingupCapture( ...
    obs, stepCount, doneParams, safetyParams);
end
